simulink library "carnot"  (R2013b)
settings: Solver=ode45  StartTime=0.0  StopTime=10.0  RelTol=1e-3
undefined symbols (not defined in the file or in its folder): A, acol, Ahabit, Awin, Azimuth_Angle, AziWin, B, C, c1, c4, capc, caph, CarnotCallbacks_Density, CarnotCallbacks_Enthalpy, CarnotCallbacks_Enthalpy2Temperature, CarnotCallbacks_Entropy, CarnotCallbacks_Evaporation_Enthalpy, CarnotCallbacks_GlobalMessageLevel, CarnotCallbacks_Grashof, CarnotCallbacks_Heat_Capacity, CarnotCallbacks_Kinematic_Viscosity, CarnotCallbacks_Prandtl, CarnotCallbacks_Saturation_Property, CarnotCallbacks_Saturation_Temperature, CarnotCallbacks_Saturation_Value_Water, CarnotCallbacks_Specific_Volume, CarnotCallbacks_Thermal_Conductivity, CarnotCallbacks_Vapour_Content, CarnotCallbacks_Vapour_Pressure, con, cond, d, Dd, density, dfin, dia, DiameterLastPiece, DPConstant, dpipe, DPLinear, DPQuadratic, emission_out, fluid, FluidMix, FluidType, FPC, frame, g, GeodeticHeight, Gwin, heat_capacity, hgt, HP, Hroom, ID, inlet, K, l, lin, lpipe ... (+29)
undefined symbols (not defined in the file): c2, c3, c5, c6, cwall, dactive, height, mc, mID, rho, tau, UAneighbour, UAwall, uloss
libraries: carnot x333, simulink x25, simulink_extras x7
(part 12 of 16)

== system carnot/Source/Solar_Thermal/Collector_Unglazed ==
  WDB : Inport
  position : Inport  Port=2
  THBin : Inport  Port=3
  Add : Sum  Inputs=1
  Bus Assignment : BusAssignment  AssignedSignals=Temperature
  Bus Selector : BusSelector  OutputSignals=Solar_Radiation_direct_surface,Solar_Radiation_diffuse_surface,Temperature_Ambient,Temperature_Sky_Radiation,Relative_Humidity,Station_Pressure,Wind_Speed  OutputAsBus=on
  Bus Selector1 : BusSelector  OutputSignals=Temperature,MassFlow,Pressure,FluidType,FluidMix  OutputAsBus=on
  IAM_Table : carnot/Source/Solar_Thermal/IncidenceAngleModifier/IAM_Table  fta=0.9  angle=[0:5:90]  Kb="[1.0000    1.0000    0.9999    0.9996    0.9991    0.9982    0.9965  0.9935    0.9886    0.9807    0.9678    0.9473    0.9148    0.8638   0.7846    0.6644    0.4907    0.2599    0.0000]"  Kd=0.92
  PowerMeter : carnot/Control/PowerMeter
  Pressure_Drop_Collector : carnot/Basic/Pressure_Drop/Pressure_Drop_Collector  len=len  lin=lin  qua=qua
  Product : Product  Inputs=*/  RndMeth=Zero
  Radiation_on_Inclined_Surface : carnot/Weather/Radiation_on_Inclined_Surface  sky=Perez 1990  reflect=0.2
  Terminator : Terminator
  Width : Width
  const : Constant  Value=acol
  create_dataC : carnot/Source/Solar_Thermal/Collector_EN12975/create_dataC
  unglazed_collector : S-Function  FunctionName=solarcollector_unglazed  Parameters=acol, uc0, uc1, uc0loss, uc1loss, uc0gain, uc1gain, e_sky, uc1eta0, hi, inv_c_abs, inv_c_fl, len, tini, nodes  EnableBusSupport=off
  Cdat : Outport
  THB : Outport  Port=2
  wires:
  unglazed_collector/3 -> Pressure_Drop_Collector/1  "Tfluid"
  Pressure_Drop_Collector/1 -> THB/1, create_dataC/3
  Width/1 -> Product/2
  Product/1 -> create_dataC/5
  Add/1 -> Product/1
  PowerMeter/1 -> create_dataC/4
  create_dataC/1 -> Cdat/1
  const/1 -> create_dataC/1
  unglazed_collector/2 -> Width/1, Add/1  "Tabsorber"
  unglazed_collector/1 -> Bus Assignment/2
  IAM_Table/2 -> Terminator/1
  Bus Selector1/1 -> unglazed_collector/3
  Bus Selector/1 -> unglazed_collector/1
  THBin/1 -> PowerMeter/2, create_dataC/2, Bus Assignment/1, Bus Selector1/1
  WDB/1 -> Radiation_on_Inclined_Surface/1
  position/1 -> Radiation_on_Inclined_Surface/2, Pressure_Drop_Collector/3
  Radiation_on_Inclined_Surface/1 -> IAM_Table/1, create_dataC/6, Bus Selector/1
  Bus Assignment/1 -> PowerMeter/1, Pressure_Drop_Collector/2
  IAM_Table/1 -> unglazed_collector/2

== system carnot/Source/Solar_Thermal/Collector_Unglazed_CONF ==
  WDB : Inport
  pos : Inport  Port=2
  THB : Inport  Port=3
  Collector_Unglazed : carnot/Source/Solar_Thermal/Collector_Unglazed  acol=USTC.Acoll  len=USTC.len  fta=USTC.fta  e_sky=USTC.eps  uc0=USTC.u0c  uc1=USTC.u1c  uc0loss=USTC.u0l  uc1loss=USTC.u1l  uc0gain=USTC.u0g  uc1gain=USTC.u1g  uc1eta0=USTC.u1e  hi=USTC.hi  c_abs=USTC.capa  c_fl=USTC.capf  lin=USTC.lin  qua=USTC.qua  tini=tini  nodes=USTC.nodes
  T_Sensor1 : carnot/Control/T_Sensor  tc=USTC.SensorTimeConstant  t0=tini
  Cdat : Outport
  Tsol : Outport  Port=2
  T'HB : Outport  Port=3
  wires:
  Collector_Unglazed/1 -> Cdat/1
  THB/1 -> Collector_Unglazed/3
  pos/1 -> Collector_Unglazed/2
  WDB/1 -> Collector_Unglazed/1
  Collector_Unglazed/2 -> T_Sensor1/1
  T_Sensor1/1 -> T'HB/1
  T_Sensor1/2 -> Tsol/1

== system carnot/Source/Solar_Thermal/IncidenceAngleModifier ==
  IAM_Table : Subsystem  mask(IAM Table for Solar Thermal Collectors){fta=0.8, angle=[0:5:90], Kb=[1.0000    1.0000    0.9999    0.9996    0.9991    0.9982    0.9965  0.9935    0.9886    0.9807    0.9678    0.9473    0.9148    0.8638   0.7846    0.6644    0.4907    0.2599    0.0000], Kd=0.92}
      mask prompts: fta "Fin Efficiency * Transmission * Absorption (FTA) [-]"; angle "Direct incidence angles for IAM [degree]"; Kb "Kdir: Incidence angle modifier direct radiation (0..1)"; Kd "Kdfu : Incidence angle modifier diffuse radiation"
      mask help:
      | Transforms direct and diffuse radiation to an absorbed solar power per unit area. The direct radiation incidence angle modifier (Kdir) uses the table-model for collectors (EN 12975).
      | FTA or F'(TauAlfa) is defined from the incidence angle modifiers Kdir and Kdfu:
      | FTA = eta0 / (Kdir(15°)*0.85 + Kdfu*0.15)
      | Direct radiation: Kdir and the incidence angle are vectors
      | Diffuse radiation  Kdfu = constant (at 50° incidence)
      mask Help: web(fullfile(path_carnot('help'),'IAM_Table.html'),'-helpbrowser')
  IAM_Table_KbL_KbT : Subsystem  mask(IAM Table for EN 12975 Solar Thermal Collector Model){fta=0.8, kblangle=[0:5:90], KbL=[1.0000    1.0000    0.9999    0.9996    0.9991    0.9982    0.9965  0.9935    0.9886    0.9807    0.9678    0.9473    0.9148    0.8638   0.7846    0.6644    0.4907    0.2599    0.0000], kbtangle=[0:5:90], KbT=[1.00000 1.00000 1.00000 1.00000 1.00000 1.00000 1.00000 1.00000 1.00000 1.00000 1.00000 0.87500 0.75000 0.62500 0.50000 0.37500 0.25000 0.12500 0], Kd=0.92}
      mask prompts: fta "Fin Efficiency * Transmission * Absorption (F'(tau alfa))"; kblangle "KbL: angles for longitudinal IAM [degree]"; KbL "KbL: values for longitudinal incidence angle modifier (0..1)"; kbtangle "KbT: angles for transversal IAM [degree]"; KbT "KbT: values for transversal incidence angle modifier (0..1)"; Kd "Kd : Incidence angle modifier diffuse radiation"
      mask help:
      | USE IN THE "Collector_EN12975" MODEL:
      | Transforms direct and diffuse radiation to an absorbed solar power per unit area. The direct radiation incidence angle modifier (Kdir) uses the b0-model for flat plate collectors (EN 12975).
      | FTA or F'(TauAlfa) is defined from the incidence angle modifiers Kdir and Kdfu:
      | FTA = eta0 / (Kdir(15°)*0.85 + Kdfu*0.15)
      | The direct radiation is split in a transversal (T) and longitudinal (L) component.
      | Direct radiation: Kb(L) and Kb(T) is given in an vecorized form
      | Diffuse radiation  Kd = constant (at 50° incidence)
      mask Help: web(fullfile(path_carnot('help'),'IAM_Table_KbL_KbT.html'),'-helpbrowser')
  IAM_b0 : Subsystem  mask(collector optics single glazing with extra white glass){fta=0.8, b0=0.12, Kd=0.92}
      mask prompts: fta "Fin Efficiency * Transmission * Absorption (FTA) [-]"; b0 "b0 : constant for the calculation of the incident angle modifier (direct radiation) [-]"; Kd "Kd : Incidence angle modifier diffuse radiation [-]"
      mask help:
      | USE IN THE "Collector_EN12975_FlatPlate" MODEL:
      | Transforms direct and diffuse radiation to an absorbed solar power per unit area. The direct radiation incidence angle modifier (Kdir) uses the b0-model for flat plate collectors (EN 12975).
      | FTA or F'(TauAlfa) is defined from the incidence angle modifiers Kdir and Kdfu:
      | FTA = eta0 / (Kdir(15°)*0.85 + Kdfu*0.15)
      mask Help: web(fullfile(path_carnot('help'),'IAM_b0.html'),'-helpbrowser')
  Theoretical_Collector_Optics : Subsystem  mask(theoretical collector optics){FTA=0.8, ncover=1, refin=1.525, d=0.004, ext=4}
      mask prompts: FTA "Fin Efficiency * Transmission * Absorption (FTA) [-]"; ncover "Number of covers [-]"; refin "Refraction index of material [-]"; d "Thickness of the material in m"; ext "Extinction coefficient in 1/m"
      mask help:
      | Transforms direct and diffuse radiation to an absorbed solar power per unit area. FTA or F'(TauAlfa) is defined from the incidence angle modifiers Kdir and Kdfu:
      | FTA = eta0 / (Kdir(15°)*0.85 + Kdfu*0.15)
      | Kdir (for direct radiation) and Kdfu (for diffuse radiation) are derived from Fresnels equations refraction index (glass = 1.526), the thickness and the extinction coefficient (extra white glass 4/m, float glass 16/m).
      | See "taualfa" in the manual or type "help taualfa" on the command line for more information on the calculation of the IAM.
      mask init:
      | teta = [0:5:90]; % incidence angle
      | KL = d*ext; % extiction * thickness
      | kb = taualfa (ncover, refin, teta*pi/180, KL, 1);
      | kd = taualfa (ncover, refin, pi/3, KL, 1);
      | kd = kd/kb(1);
      | kb = kb/kb(1);
      mask Help: web(fullfile(path_carnot('help'),'Theoretical_Collector_Optics.html'),'-helpbrowser')

== system carnot/Source/Solar_Thermal/PressureDropCollector ==
  pressure_drop_calculated_for_header_riser_water : Subsystem  mask(pressure drop for header - riser, fluid water){aonecol=1.96, acol=acol}
      mask prompts: aonecol "surface of one collector element [m²]"; acol "total surface of array (DO NOT CHANGE)"
      mask help:
      | This block interpolates the pressure drop of a collector for a usual header riser- arrangement. The number of risers (= number of absorber fins) is 10 per m². The inner diameter of the riser is 6 mm, of the header 20 mm. Fluid in the collector is water. An equation of Dunkle and Davey ("Flow distribution in absorber banks", ISES Conference, 1970) is used. See colpdrop in the manual or type "help colpdrop" on the command line for more information.
      | Set "surface of one collector" to the surface of one collector for a parallel arrangement of collectors. Set it to the surface of the array "acol" to model a series arrangement.
      mask Help: web(fullfile(path_carnot('help'),'pressure_drop_calculated_for_header_riser_water.html'),'-helpbrowser')
  pressure_drop_for_measured_data_water : Subsystem  mask(pressure drop measured data, fluid water){mdottest=0.01*1.96, ttest=20, pdroptest=158*1.96, aonecol=1.96, acol=acol}
      mask prompts: mdottest "massflow at test condition condition [kg/s]"; ttest "temperature at test condition [degree centigrade]"; pdroptest "pressure drop in test [Pa]"; aonecol "surface of one collector [m²]"; acol "total surface of array (DO NOT CHANGE HERE)"
      mask help:
      | This block calculates the pressure drop of a collector from measured data.
      | Other massflow rates and temperatures than at test condition are interpolated according to a typical massflow to pressure drop correlation of a collector for the fluid water.
      | Set "surface of one collector" to the surface of one collector for a parallel arrangement of collectors. Set it to the surface of the array "acol" to model a series arrangement.
      mask Help: web(fullfile(path_carnot('help'),'pressure_drop_for_measured_data_water.html'),'-helpbrowser')
  pressure_drop_quadratic_fitted_data : Subsystem  mask(pressure drop quadratic fitted data, fluid water){b=0.006201*3.6e4, a=0.000096*1.296e9, aonecol=1.96, acol=acol}
      mask prompts: b "linear term of pressure drop in [Pa/(kg/s)]"; a "quadratic term of pressure drop in [Pa/(kg/s)²]"; aonecol "surface of one collector element in [m²]"; acol "total surface of array (DO NOT CHANGE HERE)"
      mask help:
      | This block calculates the pressure drop of a collector from a fitted parabolic curve. Other temperatures than at test condition are not corrected.
      | Give parameters in SI-units.
      | Multiply with 3.6e5 to convert from [mbar/(l/h)] to [Pa/(kg/s)].
      | Multiply with 1.296e9 to convert from [mbar/(l/h)²] to [Pa/(kg/s)²].
      | Set "surface of one collector" to the surface of one collector for a parallel arrangement of collectors. Set it to the surface of the array "acol" to model a series arrangement.
      mask Help: web(fullfile(path_carnot('help'),'pressure_drop_quadratic_fitted_data.html'),'-helpbrowser')
  pressure_drop_quadratic_fitted_data_water : Subsystem  mask(pressure drop quadratic fitted data, fluid water){b=0.006201*3.6e4, a=0.000096*1.296e9, aonecol=1.96, acol=acol}
      mask prompts: b "linear term of pressure drop in [Pa/(kg/s)]"; a "quadratic term of pressure drop in [Pa/(kg/s)²]"; aonecol "surface of one collector element in [m²]"; acol "total surface of array (DO NOT CHANGE HERE)"
      mask help:
      | This block calculates the pressure drop of a collector from a fitted parabolic curve. Other temperatures than at test condition (20°C) are interpolated according to a typical pressure drop correlation of a collector for the fluid water.
      | Give parameters in SI-units.
      | Multiply with 3.6e5 to convert from [mbar/(l/h)] to [Pa/(kg/s)].
      | Multiply with 1.296e9 to convert from [mbar/(l/h)²] to [Pa/(kg/s)²].
      | Set "surface of one collector" to the surface of one collector for a parallel arrangement of collectors. Set it to the surface of the array "acol" to model a series arrangement.
      mask Help: web(fullfile(path_carnot('help'),'pressure_drop_quadratic_fitted_data_water.html'),'-helpbrowser')

== system carnot/Source/Ventilation/Constant_AIV ==
  const : Constant  Value=[Tsens Tcon Trad mw mco rhoair cpair pair nair]
  AIV_out : Outport
  wires:
  const/1 -> AIV_out/1

== system carnot/Source/Ventilation/Ventilation ==
  note: multiply Vhouse with
      | density and heat capacity of humid air
      | (Temperature 20°C, humidity 10 g/kg)
  Tamb : Inport
  Troom : Inport  Port=2
  Const : Constant  Value=Vhouse*vent/3600*1215*(1-rec)
  Product : Product  RndMeth=Zero
  Sum3 : Sum  Inputs=+-  SaturateOnIntegerOverflow=on  InputSameDT=on  OutDataTypeStr=Inherit: Same as first input
  Qdot_vent : Outport
  wires:
  Const/1 -> Product/1
  Product/1 -> Qdot_vent/1
  Tamb/1 -> Sum3/1
  Sum3/1 -> Product/2
  Troom/1 -> Sum3/2

== system carnot/Source/Ventilation/Ventilation_AIV ==
  note: ASSUMPTION: mdot_air_in = mdot_air_out !
  note: AIR VENTILATION outdoors - indoors
  air_exchange_rate : Inport
  "[AIV]" : Inport  Port=2
  WDB : Inport  Port=3
  Vair : Inport  Port=4
  "\"air\"" : Constant  Value=2
  "1/h -> 1/s" : Gain  Gain=1/3600  SaturateOnIntegerOverflow=on  OutDataTypeStr=Inherit: Same as input  ParamDataTypeStr=Inherit: Same as input
  Bus Selector : BusSelector  OutputSignals=Temperature_Ambient,Relative_Humidity,Station_Pressure
  Demux2 : Demux  Outputs=[1 1 1 2 4]
  Density : carnot/Basic/Material_Properties/Density  VariantControl=CarlibClassic  INPUTARGUMENTS=state variables (classic)  DEBUGLEVEL=DEBUGLEVEL  MAXTOTALWARNINGS=inf  MAXCONSECUTIVEWARNINGS=inf  WRITETOFILE=0  FILENAME='errors.txt'
  Ground10 : Ground
  Ground8 : Ground
  Heat_Capacity : carnot/Basic/Material_Properties/Heat_Capacity  VariantControl=CarlibClassic  INPUTARGUMENTS=state variables (classic)  DEBUGLEVEL=DEBUGLEVEL  MAXTOTALWARNINGS=inf  MAXCONSECUTIVEWARNINGS=inf  WRITETOFILE=0  FILENAME='errors.txt'
  Mux3 : Mux  Inputs=[5 1 1 2 1 1 1 1]
  Mux4 : Mux  Inputs=2
  Product3 : Product  Inputs=3  SaturateOnIntegerOverflow=on  InputSameDT=on  OutDataTypeStr=Inherit: Same as first input
  Product4 : Product  Inputs=3  SaturateOnIntegerOverflow=on  InputSameDT=on  OutDataTypeStr=Inherit: Same as first input
  RelHum2x : carnot/Basic/Material_Properties/RelHum2x
  Saturation : Saturate  UpperLimit=inf  LowerLimit=0
  Subsystem : Subsystem
  Sum : Sum  Inputs=-+  SaturateOnIntegerOverflow=on  InputSameDT=on  OutDataTypeStr=Inherit: Same as first input
  Terminator : Terminator
  Terminator1 : Terminator
  Terminator2 : Terminator
  rho(CO2) / rho(air) * CO2norm (kg/kg) : Constant  Value=1.529*CO2norm
  "[S]" : Outport
  wires:
  Vair/1 -> Product3/1
  Mux3/1 -> "[S]"/1
  Product4/1 -> Mux3/3, Mux3/2  "Qdot_air"
  Ground10/1 -> Mux3/1
  Ground8/1 -> Mux3/4
  Subsystem/2(mdot_CO2) -> Mux3/6  "mdot_CO2"
  Subsystem/1(mdot_H2O) -> Mux3/5  "mdot_H2O"
  WDB/1 -> Bus Selector/1
  air_exchange_rate/1 -> Saturation/1
  "[AIV]"/1 -> Demux2/1
  Density/1 -> Product3/2
  Bus Selector/3 -> RelHum2x/2, Heat_Capacity/2, Density/2  "<Station_Pressure>"
  Bus Selector/2 -> RelHum2x/3  "<Relative_Humidity>"
  Bus Selector/1 -> RelHum2x/1, Heat_Capacity/1, Density/1, Sum/2  "<Temperature_Ambient>"
  RelHum2x/1 -> Heat_Capacity/4, Density/4, Mux4/1  "x_H2O"
  "\"air\""/1 -> Heat_Capacity/3, Density/3
  Demux2/4 -> Subsystem/2(x_in)  "[x_H2O, x_CO2]_in"
  Demux2/5 -> Terminator2/1
  Demux2/3 -> Terminator1/1
  Demux2/2 -> Sum/1  "Tc"
  Mux4/1 -> Subsystem/3(x_out)
  rho(CO2) / rho(air) * CO2norm (kg/kg)/1 -> Mux4/2  "x_CO2"
  Sum/1 -> Product4/1  "dT"
  Demux2/1 -> Terminator/1
  Heat_Capacity/1 -> Product4/2  "cp"
  Product3/1 -> Product4/3, Subsystem/1(mdot_air)
  Saturation/1 -> "1/h -> 1/s"/1
  "1/h -> 1/s"/1 -> Mux3/7, Mux3/8, Product3/3

== system carnot/Source/Ventilation/Ventilation_Window ==
  note: multiply Vhouse with
      | density and heat capacity of humid air
      | (Temperature 20°C, humidity 10 g/kg)
  note: No heat recovery
      | when windows are open
  Tamb : Inport
  Troom : Inport  Port=2
  6 windows relative to Volume : Gain  Gain=6
  Constant : Constant
  Constant1 : Constant  Value=Vhouse
  Product : Product  Inputs=4  RndMeth=Zero
  Product1 : Product  Inputs=/*  RndMeth=Zero
  Sum : Sum
  Sum3 : Sum  Inputs=+-  SaturateOnIntegerOverflow=on  InputSameDT=on  OutDataTypeStr=Inherit: Same as first input
  Window_Control : carnot/Control/Window_Control
  Window_Ventilation : carnot/Basic/Ventilation/Window_Ventilation  alpha=10  H=1  W=1
  air_flow_rate : Constant  Value=vent
  heat exchange : Constant  Value=1-rec
  heat_recovery_on_off : Switch  Criteria=u2 > Threshold  Threshold=vent
  ventilation : Gain  Gain=1/3600*1215  SaturateOnIntegerOverflow=on  OutDataTypeStr=Inherit: Same as input  ParamDataTypeStr=Inherit: Same as input
  Qdot_vent : Outport
  wires:
  Window_Control/1 -> Window_Ventilation/3
  Window_Ventilation/1 -> 6 windows relative to Volume/1
  air_flow_rate/1 -> Sum/2
  Product1/1 -> Sum/1
  Troom/1 -> Sum3/2, Window_Ventilation/1, Window_Control/2
  Tamb/1 -> Sum3/1, Window_Ventilation/2, Window_Control/1
  Sum3/1 -> Product/2
  ventilation/1 -> Product/1
  Constant1/1 -> ventilation/1, Product1/1
  Product/1 -> Qdot_vent/1
  Sum/1 -> Product/3
  6 windows relative to Volume/1 -> Product1/2, heat_recovery_on_off/2
  heat exchange/1 -> heat_recovery_on_off/3
  Constant/1 -> heat_recovery_on_off/1
  heat_recovery_on_off/1 -> Product/4

== system carnot/Storage/Thermal/Ground_Storage ==
  WDB : Inport
  T_top : Inport  Port=2
  THVin : Inport  Port=3
  Tsurface : Inport  Port=4
  Tbottom : Inport  Port=5
  Demux : Demux  Outputs=[3*mpts 1 1 3]
  Demux1 : Demux  Outputs=[1 1 1 1 2 4]
  Demux2 : Demux  Outputs=[10 10]
  Isolated_Cover : carnot/Storage/Thermal/surface_models/Isolated_Cover  u=0.6
  Mux : Mux  Inputs=10
  Mux1 : Mux  Inputs=8
  Open_Surface : carnot/Storage/Thermal/surface_models/Open_Surface  albedo=0.6
  S-Function : S-Function  FunctionName=ground  Parameters=xs, ys, zs, cg, lg, dp, kp, np, zp, cf, lf, t0, refine, mpts  EnableBusSupport=off
  diameter : Constant  Value=dp
  THV : Outport
  Tnodes : Outport  Port=2
  wires:
  T_top/1 -> Isolated_Cover/1
  S-Function/1 -> Demux/1
  Demux1/1 -> Mux/3, Mux1/1  "ID"
  Isolated_Cover/1 -> Mux/2
  Open_Surface/1 -> Mux/1
  WDB/1 -> Open_Surface/1
  diameter/1 -> Mux1/6
  Mux/1 -> S-Function/1
  Demux/3 -> Mux1/4  "p"
  Demux/2 -> Mux1/2  "T"
  Mux1/1 -> THV/1
  Demux/1 -> Tnodes/1
  Tbottom/1 -> Mux/10
  Tsurface/1 -> Mux/9
  Demux1/5 -> Mux1/5, Mux/7  "fluid, mix"
  Demux1/3 -> Mux1/3, Mux/5  "mdot"
  Demux1/6 -> Mux/8  "d clq"
  Demux1/4 -> Mux/6  "p"
  Demux1/2 -> Mux/4  "T"
  THVin/1 -> Demux2/1
  Demux2/1 -> Demux1/1
  Demux2/2 -> Mux1/8
  Demux/4 -> Mux1/7  "clq"

== system carnot/Storage/Thermal/Storage_Ports ==
  Electric_Heating : Subsystem  mask(electric heating){hin=0, hout=0.4, nodes=nodes}
      mask prompts: hin "relative height start heating zone"; hout "relative height end heating zone"; nodes "Number of nodes (do not change here)"
      mask help: The block is an electric backup heating for the storage. Give inlet- and outlet-height as a relative position from 0 (= bottom) to 1 (= top).
      mask init:
      | hin = min(1, max(0, hin));
      | hout = min(1, max(0, hout));
      | 
      | if hin < hout
      |     inlet = max(ceil(hin*nodes),1);    % start node of heated zone
      |     outlet = max(ceil(hout*nodes),1);  % end node of heated zone
      | else
      |     outlet = max(ceil(hin*nodes),1);   % end node of heated zone
      |     inlet = max(ceil(hout*nodes),1);   % start node of heated zone
      | end
      | 
      | Q = zeros(nodes,1);                    % initilize power vector
      | if inlet < outlet
      |     Q(inlet:outlet) = ones(outlet-inlet+1,1); % set heated zone to One
      | else
      |     Q(outlet:inlet) = ones(inlet-outlet+1,1); % set heated zone to One
      | end
      | Q = Q./sum(Q);                         % sum over all elements must be one
      mask Help: web(fullfile(path_carnot('help'),'Electric_Heating.html'),'-helpbrowser')
  HX_EN12977 : Subsystem  mask(heat exchanger for storage, data EN 12977){h_in=0.5, h_out=0, ua0=800, uam=0, uat=0, dplin=100, dpqua=100, nodes=nodes, hgt=height, dia=dia}
      mask prompts: h_in "relative height of inlet"; h_out "relative height of outlet"; ua0 "uac: heat transfer coefficient [W/K /(kg/s) /(°C)]"; uam "uam: massflow dependent heat transfer [-]"; uat "uat: temperature difference dependent heat transfer [-]"; dplin "pressure drop linear in mdot [Pa*s/kg]"; dpqua "pressure drop quadratic in mdot [Pa*s²/kg²]"; nodes "Number of nodes (DO NOT CHANGE)"; hgt "Height vector (DO NOT CHANGE)"; dia "Diameter (DO NOT CHANGE)"
      mask help:
      | The block transforms the incoming THV vector to a vector which the storage interprets as a heat exchanger.
      | Give inlet and outlet as a relative position 0=bottom to 1=top
      | The heat transfer is calculated by:
      | UA = uac * mdot^uam * ((Theatexchanger+Tstorage)/2)^uat
      mask init:
      | in = zeros(nodes,1);    % vector of length nodes
      | up = in;                % vector of length nodes
      | down = in;              % vector of length nodes
      | 
      | h_in = max(0,h_in);     % no nodes below 0
      | h_out = max(0,h_out);   % no nodes below 0
      | 
      | inlet = round(h_in*(nodes-1))+1;    % inlet position
      | outlet = round(h_out*(nodes-1))+1;  % outlet position
      | hgt = (h_out-h_in)*hgt;
      | 
      | in(inlet)=1;
      | 
      | if (h_in < h_out)           % if inlet below outlet
      |     up(inlet:outlet)=1;     % upwards
      | elseif (h_in > h_out)       % else if inlet above outlet
      |     down(outlet:inlet)=1;   % downwards
      | end
      mask Help: web(['file:///' fullfile(path_carnot('help'),'StoragePorts_HeatExchangerModels.html')],'-helpbrowser')
      mask Display: disp('HX EN12977')
  HX_EN12977_stratified : Subsystem  mask(stratified heat exchanger for storage, data EN 12977){h_in=1, h_out=0, ua0=800, uam=0, uat=0, dplin=100, dpqua=100, nodes=nodes, hgt=height, dia=dia}
      mask prompts: h_in "relative height of inlet"; h_out "relative height of outlet"; ua0 "uac: heat transfer coefficient [W/K /(kg/s) /(°C)]"; uam "uam: massflow dependent heat transfer [-]"; uat "uat: temperature difference dependent heat transfer [-]"; dplin "pressure drop linear in mdot [Pa*s/kg]"; dpqua "pressure drop quadratic in mdot [Pa*s²/kg²]"; nodes "Number of nodes (DO NOT CHANGE)"; hgt "Height vector (DO NOT CHANGE)"; dia "Diameter (DO NOT CHANGE)"
      mask help:
      | The block transforms the incoming THV vector to a vector which the storage interprets as a heat exchanger.
      | Give inlet and outlet as a relative position 0=bottom to 1=top
      | The heat transfer is calculated by:
      | UA = uac * mdot^uam * ((Theatexchanger+Tstorage)/2)^uat
      |
      | Stratified:
      | For charging (inlet above outlet) the heat transfer starts when the storage temperature is below the heat exchanger temperature.
      | For discharging (outlet above inlet) the heat transfer starts when the storage temperature is above the heat exchanger temperature.
      mask init: same as carnot/Storage/Thermal/Storage_Ports/HX_EN12977
      mask Help: web(['file:///' fullfile(path_carnot('help'),'StoragePorts_HeatExchangerModels.html')],'-helpbrowser')
      mask Display: disp('HX EN12977 STRAT')
  HX_data_fit : Subsystem  mask(heat exchanger for storage, fitted data){h_in=1, h_out=0, ua0=800, uam=0, uat=0, dplin=100, dpqua=100, nodes=nodes, hgt=height, dia=dia}
      mask prompts: h_in "relative height of inlet"; h_out "relative height of outlet"; ua0 "uac: constant heat transfer coefficient [W/K]"; uam "uam: massflow dependent heat transfer [W*s/(K*kg)]"; uat "uat: temperature difference dependent heat transfer [W/K²]"; dplin "pressure drop linear in mdot [Pa*s/kg]"; dpqua "pressure drop quadratic in mdot [Pa*s²/kg²]"; nodes "Number of nodes (DO NOT CHANGE)"; hgt "Height vector (DO NOT CHANGE)"; dia "Diameter (DO NOT CHANGE)"
      mask help:
      | The block transforms the incoming THV vector to a vector which the storage interprets as a heat exchanger.
      | Give inlet and outlet as a relative position 0=bottom to 1=top
      | The heat transfer is calculated by:
      | UA = uac + mdot*uam + (Theatexchanger-Tstorage)*uat
      mask init:
      | in = zeros(nodes,1);    % vector of length nodes
      | up = in;                % vector of length nodes
      | down = in;              % vector of length nodes
      | 
      | h_in = max(0,h_in);     % no nodes below 0
      | h_out = max(0,h_out);   % no nodes below 0
      | 
      | inlet = round(h_in*(nodes-1))+1;    % inlet position
      | outlet = round(h_out*(nodes-1))+1;  % outlet position
      | hgt = (h_out-h_in)*hgt;
      | in(inlet)=1;
      | 
      | if (h_in < h_out)           % if inlet below outlet
      |     up(inlet:outlet)=1;     % upwards
      | elseif (h_in > h_out)       % else if inlet above outlet
      |     down(outlet:inlet)=1;   % downwards
      | end
      mask Help: web(fullfile(path_carnot('help'),'StoragePorts_HeatExchangerModels.html'),'-helpbrowser')
      mask Display: disp('HX data')
  HX_data_fit_stratified : Subsystem  mask(stratified heat exchanger for storage, fitted data){h_in=1, h_out=0, ua0=800, uam=0, uat=0, dplin=100, dpqua=100, nodes=nodes, hgt=height, dia=dia}
      mask prompts: h_in "relative height of inlet"; h_out "relative height of outlet"; ua0 "uac: constant heat transfer coefficient [W/K]"; uam "uam: massflow dependent heat transfer [W*s/(K*kg)]"; uat "uat: temperature difference dependent heat transfer [W/K²]"; dplin "pressure drop linear in mdot [Pa*s/kg]"; dpqua "pressure drop quadratic in mdot [Pa*s²/kg²]"; nodes "Number of nodes (DO NOT CHANGE)"; hgt "Height vector (DO NOT CHANGE)"; dia "Diameter (DO NOT CHANGE)"
      mask help:
      | The block transforms the incoming THV vector to a vector which the storage interprets as a heat exchanger.
      | Give inlet and outlet as a relative position 0=bottom to 1=top
      | The heat transfer is calculated by:
      | UA = uac + mdot*uam + (Theatexchanger-Tstorage)*uat
      |
      | Stratified:
      | For charging (inlet above outlet) the heat transfer starts when the storage temperature is below the heat exchanger temperature.
      | For discharging (outlet above inlet) the heat transfer starts when the storage temperature is above the heat exchanger temperature.
      mask init: same as carnot/Storage/Thermal/Storage_Ports/HX_EN12977
      mask Help: web(['file:///' fullfile(path_carnot('help'),'StoragePorts_HeatExchangerModels.html')],'-helpbrowser')
      mask Display: disp('HX data STRAT')
  HX_finned_tube : Subsystem  mask(finned tube heat exchanger for storage){h_in=0.5, h_out=0, dpipe=0.03, swall=0.002, lpipe=15, cond=50, dfin=0.05, sfin=0.001, nfin=100, dplin=100, dpqua=100, nodes=nodes, hgt=height, dia=dia}
      mask prompts: h_in "relative height of inlet"; h_out "relative height of outlet"; dpipe "outer diameter of HX pipe in m (without fins)"; swall "thickness of pipe wall in m"; lpipe "length of HX pipe in m"; cond "thermal conductivity of HX wall in W/m/K"; dfin "diameter of HX pipe with fins in m"; sfin "wall thickness of fins in m"; nfin "number of fins per length in 1/m"; dplin "pressure drop linear in mdot [Pa*s/kg]"; dpqua "pressure drop quadratic in mdot [Pa*s²/kg²]"; nodes "Number of nodes (DO NOT CHANGE)"; hgt "Height vector (DO NOT CHANGE)"; dia "Diameter (DO NOT CHANGE)"
      mask help:
      | The block transforms the incoming THV vector to a vector which the storage interprets as a heat exchanger.
      | Give inlet and outlet as a relative position 0=bottom to 1=top
      | The heat transfer is calculated by a theoretical equation from Wagner: Waermeuebertragung, Vogel Fachbuch, 1991
      mask init:
      | in = zeros(nodes,1);    % vector of length nodes
      | up = in;                % vector of length nodes
      | down = in;              % vector of length nodes
      | 
      | h_in = max(0,h_in);     % no nodes below 0
      | h_out = max(0,h_out);   % no nodes below 0
      | hgt = (h_out-h_in)*hgt;
      | 
      | inlet = round(h_in*(nodes-1))+1;    % inlet position
      | outlet = round(h_out*(nodes-1))+1;  % outlet position
      | 
      | in(inlet)=1;
      | 
      | if (h_in < h_out)           % if inlet below outlet
      |     up(inlet:outlet)=1;     % upwards
      | elseif (h_in > h_out)       % else if inlet above outlet
      |     down(outlet:inlet)=1;   % downwards
      | end
      | 
      | dfin = max(dfin,dpipe);
      | nfin = max(nfin, 0);
      | if (sfin < 1e-5)
      |    sfin = 1e-5;
      |    disp('fin width set to minimum 0.01 mm')
      | end
      mask Help: web(['file:///' fullfile(path_carnot('help'),'StoragePorts_HeatExchangerModels.html')],'-helpbrowser')
      mask Display: disp('HX finned tube')
  HX_finned_tube_stratified : Subsystem  mask(stratified finned tube heat exchanger for storage){h_in=1, h_out=0, dpipe=0.03, swall=0.002, lpipe=15, cond=50, dfin=0.05, sfin=0.001, nfin=100, dplin=100, dpqua=100, nodes=nodes, hgt=height, dia=dia}
      mask prompts: h_in "relative height of inlet"; h_out "relative height of outlet"; dpipe "outer diameter of HX pipe in m (without fins)"; swall "thickness of pipe wall in m"; lpipe "length of HX pipe in m"; cond "thermal conductivity of HX wall in W/m/K"; dfin "diameter of HX pipe with fins in m"; sfin "wall thickness of fins in m"; nfin "number of fins per length in 1/m"; dplin "pressure drop linear in mdot [Pa*s/kg]"; dpqua "pressure drop quadratic in mdot [Pa*s²/kg²]"; nodes "Number of nodes (DO NOT CHANGE)"; hgt "Height vector (DO NOT CHANGE)"; dia "Diameter (DO NOT CHANGE)"
      mask help:
      | The block transforms the incoming THV vector to a vector which the storage interprets as a heat exchanger.
      | Give inlet and outlet as a relative position 0=bottom to 1=top
      | The heat transfer is calculated by a theoretical equation from Wagner: Waermeuebertragung, Vogel Fachbuch, 1991
      |
      | Stratified:
      | For charging (inlet above outlet) the heat transfer starts when the storage temperature is below the heat exchanger temperature.
      | For discharging (outlet above inlet) the heat transfer starts when the storage temperature is above the heat exchanger temperature.
      mask init: same as carnot/Storage/Thermal/Storage_Ports/HX_finned_tube
      mask Help: web(['file:///' fullfile(path_carnot('help'),'StoragePorts_HeatExchangerModels.html')],'-helpbrowser')
      mask Display: disp('HX finned tube STRAT')
  HX_tube : Subsystem  mask(smooth tube heat exchanger for storage){h_in=0.5, h_out=0, dpipe=0.03, swall=0.002, lpipe=15, cond=50, dplin=100, dpqua=100, nodes=nodes, hgt=height, dia=dia}
      mask prompts: h_in "relative height of inlet"; h_out "relative height of outlet"; dpipe "outer diameter of HX pipe in m"; swall "thickness of pipe wall in m"; lpipe "length of HX pipe in m"; cond "thermal conductivity of HX wall in W/m/K"; dplin "pressure drop linear in mdot [Pa*s/kg]"; dpqua "pressure drop quadratic in mdot [Pa*s²/kg²]"; nodes "Number of nodes (DO NOT CHANGE)"; hgt "Height vector (DO NOT CHANGE)"; dia "Diameter (DO NOT CHANGE)"
      mask help:
      | The block transforms the incoming THV vector to a vector which the storage interprets as a heat exchanger.
      | Give inlet and outlet as a relative position 0=bottom to 1=top
      | The heat transfer is calculated with an equation from Wagner: Waermeuebertragung, Vogel-Verlag, 1991
      mask init: same as carnot/Storage/Thermal/Storage_Ports/HX_EN12977
      mask Help: web(['file:///' fullfile(path_carnot('help'),'StoragePorts_HeatExchangerModels.html')],'-helpbrowser')
      mask Display: disp('HX tube')
  HX_tube_stratified : Subsystem  mask(stratified smooth tube heat exchanger for storage){h_in=1, h_out=0, dpipe=0.03, swall=0.002, lpipe=15, cond=50, dplin=100, dpqua=100, nodes=nodes, hgt=height, dia=dia}
      mask prompts: h_in "relative height of inlet"; h_out "relative height of outlet"; dpipe "outer diameter of HX pipe in m"; swall "thickness of pipe wall in m"; lpipe "length of HX pipe in m"; cond "thermal conductivity of HX wall in W/m/K"; dplin "pressure drop linear in mdot [Pa*s/kg]"; dpqua "pressure drop quadratic in mdot [Pa*s²/kg²]"; nodes "Number of nodes (DO NOT CHANGE)"; hgt "Height vector (DO NOT CHANGE)"; dia "Diameter (DO NOT CHANGE)"
      mask help:
      | The block transforms the incoming THV vector to a vector which the storage interprets as a heat exchanger.
      | Give inlet and outlet as a relative position 0=bottom to 1=top
      | The heat transfer is calculated with an equation from Wagner: Waermeuebertragung, Vogel-Verlag, 1991
      |
      | Stratified:
      | For charging (inlet above outlet) the heat transfer starts when the storage temperature is below the heat exchanger temperature.
      | For discharging (outlet above inlet) the heat transfer starts when the storage temperature is above the heat exchanger temperature.
      mask init: same as carnot/Storage/Thermal/Storage_Ports/HX_EN12977
      mask Help: web(['file:///' fullfile(path_carnot('help'),'StoragePorts_HeatExchangerModels.html')],'-helpbrowser')
      mask Display: disp('HX tube STRAT')
  Pipe : Subsystem  mask(pipe connection to storage){h_in=0, h_out=1, nodes=nodes, hgt=height, dia=dia, dplin=0, dpqua=0}
      mask prompts: h_in "relative height of inlet"; h_out "relative height of outlet"; nodes "Number of nodes of storage (DO NOT CHANGE)"; hgt "Height vector (DO NOT CHANGE)"; dia "Diameter (DO NOT CHANGE)"; dplin "linear pressure drop"; dpqua "quadratic pressure drop"
      mask help:
      | The block transforms the incoming THV vector to a vector which the storage interprets as a flow into the storage fluid.
      | Give inlet- and outlet-height as a relative position from 0 (= bottom) to 1 (= top).
      mask init:
      | in = zeros(nodes,1);    % vector of length nodes
      | up = in;                % vector of length nodes
      | down = in;              % vector of length nodes
      | 
      | h_in = max(0,min(h_in,1));     % no nodes below 0
      | h_out = max(0,min(h_out,1));   % no nodes below 0
      | hgt = (h_out-h_in)*hgt;
      |  
      | inlet = max(ceil(h_in*nodes),1);    % inlet position
      | outlet = max(ceil(h_out*nodes),1);  % outlet position
      |  
      | in(inlet)=1;
      |  
      | idx_in_out = inlet:outlet;
      | if (inlet < outlet)         % if inlet below outlet
      |     up(inlet:outlet-1)=1;   % upwards
      | elseif (inlet > outlet)     % else if inlet above outlet
      |     down(outlet:inlet-1)=1; % downwards
      |     idx_in_out = outlet:inlet;
      | end
      mask Help: web(fullfile(path_carnot('help'),'StoragePorts_PipeConnections.html'),'-helpbrowser')
      mask Display: disp('Pipe')
  Pipe_stratified : Subsystem  mask(pipe connection to storage){h_in=0, h_out=0.8, nodes=nodes, hgt=height, dia=dia, dplin=0, dpqua=0}
      mask prompts: h_in "relative height of inlet"; h_out "relative height of outlet"; nodes "Number of nodes of storage (DO NOT CHANGE)"; hgt "Height vector (DO NOT CHANGE)"; dia "Diameter (DO NOT CHANGE)"; dplin "linear pressure drop"; dpqua "quadratic pressure drop"
      mask help:
      | The block transforms the incoming THV vector to a vector which the storage interprets as a flow into the storage fluid.
      | Give inlet- and outlet-height as a relative position from 0 (= bottom) to 1 (= top).
      mask init:
      | in = zeros(nodes,1);    % vector of length nodes
      | up = in;                % vector of length nodes
      | down = in;              % vector of length nodes
      | 
      | h_in = max(0,min(h_in,1));     % no nodes below 0 and above 1
      | h_out = max(0,min(h_out,1));   % no nodes below 0 and above 1
      | 
      | inlet = max(ceil(h_in*nodes),1);    % inlet position
      | outlet = max(ceil(h_out*nodes),1);  % outlet position
      | hgt = (h_out-h_in)*hgt;
      | 
      | in(inlet)=1;
      | 
      | 
      | idx_in_out = inlet:outlet;
      | if (inlet < outlet)             % if inlet below outlet
      |     up(inlet:outlet-1)=1;       % upwards
      |     n_concerned = inlet:outlet;
      |     flowdir = 1;
      | elseif (inlet > outlet)         % else if inlet above outlet
      |     down(outlet:inlet-1)=1;     % downwards
      |     n_concerned = outlet:inlet;
      |     idx_in_out = outlet:inlet;
      |     flowdir = -1;
      | end
      mask Help: web(fullfile(path_carnot('help'),'StoragePorts_PipeConnections.html'),'-helpbrowser')
      mask Display: disp('Pipe STRAT')

== system carnot/Storage/Thermal/Storage_Type_1 ==
  Tamb : Inport
  THB_chg : Inport  Port=2
  THB_dis : Inport  Port=3
  Bus Creator : BusCreator  Inputs=13
  Bus Creator1 : BusCreator  Inputs=2
  Demux : Demux  Outputs=2
  constant_THB{,1,6..9} (6 alike) : carnot/Source/Simple/Constant_THB  t=20  mdot=0  p=1e5  mID=No Pressure Drop  fluid=Water  mix=0  dia=0.02  hgt=0
  pipe_charge : carnot/Storage/Thermal/Storage_Ports/Pipe  h_in=1  h_out=0  nodes=nodes  hgt=height  dia=dia  dplin=10  dpqua=10
  pipe_discharge : carnot/Storage/Thermal/Storage_Ports/Pipe  h_in=0  h_out=1  nodes=nodes  hgt=height  dia=dia  dplin=10  dpqua=10
  select_T : Selector  InputPortWidth=nodes  IndexOptions=Index vector (dialog)  Indices=mpts  OutputSizes=1
  sfun_storageTnodes : carnot/Basic/Thermal_Models/sfun_storageTnodes  dia=dia  volume=volume  standing=standing  uloss=uloss  ubot=utop  utop=ubot  cond=cond  tini=tini  nodes=nodes  nconnect=nconnect
  Sdat : Outport
  T_nodes : Outport  Port=2
  THBchg : Outport  Port=3
  THBdis : Outport  Port=4
  wires:
  Tamb/1 -> sfun_storageTnodes/1, Bus Creator/1  "Tamb"
  THB_dis/1 -> pipe_discharge/2, Bus Creator/5  "THBheating_in"
  pipe_discharge/2 -> THBdis/1, Bus Creator/6  "THBheating_out"
  pipe_discharge/1 -> sfun_storageTnodes/2
  select_T/1 -> T_nodes/1, Bus Creator/13  "Tnodes"
  sfun_storageTnodes/1 -> Demux/1  "Energy"
  sfun_storageTnodes/2 -> select_T/1, pipe_charge/1, pipe_discharge/1  "Tnodes"
  constant_THB1/1 -> Bus Creator/4  "THBdhw_out"
  constant_THB/1 -> Bus Creator/3  "THBdhw_in"
  Bus Creator/1 -> Sdat/1
  constant_THB9/1 -> Bus Creator/12  "THBsolar_out"
  constant_THB8/1 -> Bus Creator/11  "THBsolar_in"
  constant_THB7/1 -> Bus Creator/10  "THBother_out"
  constant_THB6/1 -> Bus Creator/9  "THBother_in"
  THB_chg/1 -> pipe_charge/2, Bus Creator/7  "THBbackup_in"
  pipe_charge/2 -> THBchg/1, Bus Creator/8  "THBbackup_out"
  pipe_charge/1 -> sfun_storageTnodes/3
  Demux/1 -> Bus Creator1/1  "internal"
  Demux/2 -> Bus Creator1/2  "losses"
  Bus Creator1/1 -> Bus Creator/2  "energy"

== system carnot/Storage/Thermal/Storage_Type_1_CONF ==
  Tamb : Inport
  THB_chg : Inport  Port=2
  THB_dis : Inport  Port=3
  Storage_Type_1 : carnot/Storage/Thermal/Storage_Type_1  uloss=1  ubot=1  utop=1  cond=1  t0=tini  volume=0.3  dia=0.5  pos=standing cylinder  nconnect=2  nodes=10  mpoints=10
  T_Sensor_Surface : carnot/Control/T_Sensor_Surface  pos=[0.5]  tdel=10  t0=tini(1)
  Sdat : Outport
  Tstg : Outport  Port=2
  THBchg : Outport  Port=3
  THBdis : Outport  Port=4
  wires:
  T_Sensor_Surface/1 -> Tstg/1
  Tamb/1 -> Storage_Type_1/1
  THB_chg/1 -> Storage_Type_1/2
  THB_dis/1 -> Storage_Type_1/3
  Storage_Type_1/1 -> Sdat/1
  Storage_Type_1/2 -> T_Sensor_Surface/1
  Storage_Type_1/3 -> THBchg/1
  Storage_Type_1/4 -> THBdis/1

== system carnot/Storage/Thermal/Storage_Type_2 ==
  Tamb : Inport
  THB_dhw : Inport  Port=2
  THB_bkp : Inport  Port=3
  Bus Creator : BusCreator  Inputs=13
  Bus Creator1 : BusCreator  Inputs=2
  Demux : Demux  Outputs=2
  HX_data_fit : carnot/Storage/Thermal/Storage_Ports/HX_data_fit  h_in=0.5  h_out=0.1  ua0=80  uam=0.2  uat=0.5  dplin=100  dpqua=100  nodes=nodes  hgt=height  dia=dia
  constant_THB{2..3,6..9} (6 alike) : carnot/Source/Simple/Constant_THB  t=20  mdot=0  p=1e5  mID=No Pressure Drop  fluid=Water  mix=0  dia=0.02  hgt=0
  pipe : carnot/Storage/Thermal/Storage_Ports/Pipe  h_in=0  h_out=1  nodes=nodes  hgt=height  dia=dia  dplin=10  dpqua=10
  select_T : Selector  InputPortWidth=nodes  IndexOptions=Index vector (dialog)  Indices=mpts  OutputSizes=1
  sfun_storageTnodes : carnot/Basic/Thermal_Models/sfun_storageTnodes  dia=dia  volume=volume  standing=standing  uloss=uloss  ubot=utop  utop=ubot  cond=cond  tini=tini  nodes=nodes  nconnect=nconnect
  Sdat : Outport
  T_nodes : Outport  Port=2
  THBdhw : Outport  Port=3
  THBbkp : Outport  Port=4
  wires:
  Bus Creator1/1 -> Bus Creator/2  "energy"
  Demux/2 -> Bus Creator1/2  "losses"
  Demux/1 -> Bus Creator1/1  "internal"
  HX_data_fit/1 -> sfun_storageTnodes/3
  HX_data_fit/2 -> THBbkp/1, Bus Creator/8  "THBbackup_out"
  THB_bkp/1 -> HX_data_fit/2, Bus Creator/7  "THBbackup_in"
  constant_THB3/1 -> Bus Creator/6  "THBheating_out"
  constant_THB2/1 -> Bus Creator/5  "THBheating_in"
  constant_THB6/1 -> Bus Creator/9  "THBother_in"
  constant_THB7/1 -> Bus Creator/10  "THBother_out"
  constant_THB8/1 -> Bus Creator/11  "THBsolar_in"
  constant_THB9/1 -> Bus Creator/12  "THBsolar_out"
  Bus Creator/1 -> Sdat/1
  sfun_storageTnodes/2 -> HX_data_fit/1, pipe/1, select_T/1  "T_d_c"
  sfun_storageTnodes/1 -> Demux/1  "Energy"
  select_T/1 -> Bus Creator/13, T_nodes/1  "Tnodes"
  pipe/1 -> sfun_storageTnodes/2
  pipe/2 -> THBdhw/1, Bus Creator/4  "THBdhw_out"
  THB_dhw/1 -> pipe/2, Bus Creator/3  "THBdhw_in"
  Tamb/1 -> Bus Creator/1, sfun_storageTnodes/1  "Tamb"

== system carnot/Storage/Thermal/Storage_Type_2_CONF ==
  Tamb : Inport
  THB_dhw : Inport  Port=2
  THB_bkp : Inport  Port=3
  Storage_Type_2 : carnot/Storage/Thermal/Storage_Type_2  uloss=1  ubot=1  utop=1  cond=1  t0=tini  volume=0.3  dia=0.5  pos=standing cylinder  nconnect=2  nodes=10  mpoints=10
  T_Sensor_Surface : carnot/Control/T_Sensor_Surface  pos=[0.5]  tdel=10  t0=tini(1)
  Sdat : Outport
  Tstg : Outport  Port=2
  THBdhw : Outport  Port=3
  THBbkp : Outport  Port=4
  wires:
  T_Sensor_Surface/1 -> Tstg/1
  Storage_Type_2/4 -> THBbkp/1
  Storage_Type_2/3 -> THBdhw/1
  Storage_Type_2/2 -> T_Sensor_Surface/1
  Storage_Type_2/1 -> Sdat/1
  THB_bkp/1 -> Storage_Type_2/3  "THBbackup_in"
  THB_dhw/1 -> Storage_Type_2/2  "THBdhw_in"
  Tamb/1 -> Storage_Type_2/1

== system carnot/Storage/Thermal/Storage_Type_3 ==
  Tamb : Inport
  THB_dhw : Inport  Port=2
  THB_bkp : Inport  Port=3
  THB_solar : Inport  Port=4
  Bus Creator : BusCreator  Inputs=13
  Bus Creator1 : BusCreator  Inputs=2
  Demux : Demux  Outputs=2
  HX_EN12977_bkp : carnot/Storage/Thermal/Storage_Ports/HX_EN12977  h_in=0.81  h_out=0.56  ua0=80  uam=0.2  uat=0.5  dplin=100  dpqua=100  nodes=nodes  hgt=height  dia=dia
  HX_EN12977_solar : carnot/Storage/Thermal/Storage_Ports/HX_EN12977  h_in=0.48  h_out=0.04  ua0=100  uam=0.2  uat=0.5  dplin=100  dpqua=100  nodes=nodes  hgt=height  dia=dia
  constant_THB{2..3,6..7} (4 alike) : carnot/Source/Simple/Constant_THB  t=20  mdot=0  p=1e5  mID=No Pressure Drop  fluid=Water  mix=0  dia=0.02  hgt=0
  pipe : carnot/Storage/Thermal/Storage_Ports/Pipe  h_in=0  h_out=1  nodes=nodes  hgt=height  dia=dia  dplin=10  dpqua=10
  select_T : Selector  InputPortWidth=nodes  IndexOptions=Index vector (dialog)  Indices=mpts  OutputSizes=1
  sfun_storageTnodes : carnot/Basic/Thermal_Models/sfun_storageTnodes  dia=dia  volume=volume  standing=standing  uloss=uloss  ubot=utop  utop=ubot  cond=cond  tini=tini  nodes=nodes  nconnect=nconnect
  Sdat : Outport
  T_nodes : Outport  Port=2
  THBdhw : Outport  Port=3
  THBbkp : Outport  Port=4
  THBsolar : Outport  Port=5
  wires:
  Tamb/1 -> sfun_storageTnodes/1, Bus Creator/1  "Tamb"
  THB_dhw/1 -> pipe/2, Bus Creator/3  "THBdhw_in"
  pipe/2 -> THBdhw/1, Bus Creator/4  "THBdhw_out"
  pipe/1 -> sfun_storageTnodes/2
  select_T/1 -> T_nodes/1, Bus Creator/13  "Tnodes"
  sfun_storageTnodes/1 -> Demux/1  "Energy"
  sfun_storageTnodes/2 -> select_T/1, pipe/1, HX_EN12977_bkp/1, HX_EN12977_solar/1  "T_d_c"
  Bus Creator/1 -> Sdat/1
  constant_THB7/1 -> Bus Creator/10  "THBother_out"
  constant_THB6/1 -> Bus Creator/9  "THBother_in"
  constant_THB2/1 -> Bus Creator/5  "THBheating_in"
  constant_THB3/1 -> Bus Creator/6  "THBheating_out"
  THB_bkp/1 -> HX_EN12977_bkp/2, Bus Creator/7  "THBbackup_in"
  HX_EN12977_bkp/2 -> THBbkp/1, Bus Creator/8  "THBbackup_out"
  HX_EN12977_bkp/1 -> sfun_storageTnodes/3
  Demux/1 -> Bus Creator1/1  "internal"
  Demux/2 -> Bus Creator1/2  "losses"
  Bus Creator1/1 -> Bus Creator/2  "energy"
  HX_EN12977_solar/1 -> sfun_storageTnodes/4
  THB_solar/1 -> HX_EN12977_solar/2, Bus Creator/11  "THBsolar_in"
  HX_EN12977_solar/2 -> THBsolar/1, Bus Creator/12  "THBsolar_out"

== system carnot/Storage/Thermal/Storage_Type_3_CONF ==
  Tamb : Inport
  THB_dhw : Inport  Port=2
  THB_bkp : Inport  Port=3
  THB_solar : Inport  Port=4
  Storage_Type_3 : carnot/Storage/Thermal/Storage_Type_3  uloss=1  ubot=1  utop=1  cond=1  t0=tini  volume=0.3  dia=0.5  pos=standing cylinder  nconnect=3  nodes=10  mpoints=10
  T_Sensor_Surface : carnot/Control/T_Sensor_Surface  pos="[0.1         0.7]"  tdel=10  t0=tini(1)
  Sdat : Outport
  Tstg : Outport  Port=2
  THBdhw : Outport  Port=3
  THBbkp : Outport  Port=4
  THBsolar : Outport  Port=5
  wires:
  T_Sensor_Surface/1 -> Tstg/1
  Tamb/1 -> Storage_Type_3/1
  THB_dhw/1 -> Storage_Type_3/2  "THBdhw_in"
  THB_bkp/1 -> Storage_Type_3/3  "THBbackup_in"
  THB_solar/1 -> Storage_Type_3/4  "THBsolar_in"
  Storage_Type_3/1 -> Sdat/1
  Storage_Type_3/2 -> T_Sensor_Surface/1
  Storage_Type_3/3 -> THBdhw/1
  Storage_Type_3/4 -> THBbkp/1
  Storage_Type_3/5 -> THBsolar/1

== system carnot/Storage/Thermal/Storage_Type_4 ==
  Tamb : Inport
  THB_dhw : Inport  Port=2
  THB_bkDHW : Inport  Port=3
  THB_heating : Inport  Port=4
  THB_solar : Inport  Port=5
  Bus Creator : BusCreator  Inputs=13
  Bus Creator1 : BusCreator  Inputs=2
  Demux : Demux  Outputs=2
  HX_EN12977_dhw : carnot/Storage/Thermal/Storage_Ports/HX_EN12977  h_in=0.02  h_out=0.95  ua0=642.2  uam=0.369  uat=0.684  dplin=100  dpqua=100  nodes=nodes  hgt=height  dia=dia
  HX_EN12977_solar : carnot/Storage/Thermal/Storage_Ports/HX_EN12977  h_in=0.45  h_out=0  ua0=678.6  uam=0.411  uat=0.287  dplin=100  dpqua=100  nodes=nodes  hgt=height  dia=dia
  constant_THB6 : carnot/Source/Simple/Constant_THB  t=20  mdot=0  p=1e5  mID=No Pressure Drop  fluid=Water  mix=0  dia=0.02  hgt=0
  constant_THB7 : carnot/Source/Simple/Constant_THB  t=20  mdot=0  p=1e5  mID=No Pressure Drop  fluid=Water  mix=0  dia=0.02  hgt=0
  pipe_bkp_dhw : carnot/Storage/Thermal/Storage_Ports/Pipe  h_in=1  h_out=0.54  nodes=nodes  hgt=height  dia=dia  dplin=10  dpqua=10
  pipe_heating : carnot/Storage/Thermal/Storage_Ports/Pipe  h_in=0.45  h_out=0.54  nodes=nodes  hgt=height  dia=dia  dplin=10  dpqua=10
  select_T : Selector  InputPortWidth=nodes  IndexOptions=Index vector (dialog)  Indices=mpts  OutputSizes=1
  sfun_storageTnodes : carnot/Basic/Thermal_Models/sfun_storageTnodes  dia=dia  volume=volume  standing=standing  uloss=uloss  ubot=utop  utop=ubot  cond=cond  tini=tini  nodes=nodes  nconnect=nconnect
  Sdat : Outport
  T_nodes : Outport  Port=2
  THBdhw : Outport  Port=3
  THBbkDHW : Outport  Port=4
  THBheating : Outport  Port=5
  THBsolar : Outport  Port=6
  wires:
  HX_EN12977_solar/2 -> Bus Creator/12, THBsolar/1  "THBsolar_out"
  THB_solar/1 -> Bus Creator/11, HX_EN12977_solar/2  "THBsolar_in"
  Bus Creator1/1 -> Bus Creator/2  "energy"
  Demux/2 -> Bus Creator1/2  "losses"
  Demux/1 -> Bus Creator1/1  "internal"
  pipe_bkp_dhw/1 -> sfun_storageTnodes/3
  pipe_bkp_dhw/2 -> THBbkDHW/1, Bus Creator/10  "THBother_out"
  THB_bkDHW/1 -> pipe_bkp_dhw/2, Bus Creator/9  "THBother_in"
  Bus Creator/1 -> Sdat/1
  sfun_storageTnodes/2 -> pipe_bkp_dhw/1, HX_EN12977_solar/1, pipe_heating/1, HX_EN12977_dhw/1, select_T/1  "T_d_c"
  sfun_storageTnodes/1 -> Demux/1  "Energy"
  select_T/1 -> Bus Creator/13, T_nodes/1  "Tnodes"
  HX_EN12977_dhw/1 -> sfun_storageTnodes/2
  HX_EN12977_dhw/2 -> Bus Creator/4, THBdhw/1  "THBdhw_out"
  THB_dhw/1 -> Bus Creator/3, HX_EN12977_dhw/2  "THBdhw_in"
  Tamb/1 -> Bus Creator/1, sfun_storageTnodes/1  "Tamb"
  THB_heating/1 -> pipe_heating/2, Bus Creator/5  "THBheating_in"
  pipe_heating/1 -> sfun_storageTnodes/4
  HX_EN12977_solar/1 -> sfun_storageTnodes/5
  pipe_heating/2 -> THBheating/1, Bus Creator/6  "THBheating_out"
  constant_THB6/1 -> Bus Creator/7  "THBbackup_in"
  constant_THB7/1 -> Bus Creator/8  "THBbackup_out"
